simulink model "landing_model"  (R2025b)
settings: Solver=ode4  StartTime=0.0  StopTime=400  FixedStep=0.001  RelTol=1e-3
values from neighbouring files (symbols this model uses):
  a0 = 340.294    [basedata.m]    (also in basedata.mat; control_design.mat; landing_init.m; landing_plan.mat)
  b_ref = 2.0    (= 2)    [basedata.m]    (also in basedata.mat; control_design.mat; landing_init.m; landing_plan.mat)
  c_gear = [0.8e4, 1.4e4, 1.4e4]    [basedata.m]    (also in basedata.mat = [8000 14000 14000]; control_design.mat = [8000 14000 14000]; landing_init.m; landing_plan.mat = [8000 14000 14000])
  c_lat = [1.4e4, 2.2e4, 2.2e4]    [basedata.m]    (also in basedata.mat = [14000 22000 22000]; control_design.mat = [14000 22000 22000]; landing_init.m; landing_plan.mat = [14000 22000 22000])
  c_ref = 0.9    [basedata.m]    (also in basedata.mat; control_design.mat; landing_init.m; landing_plan.mat)
  c_roll = [0.020, 0.018, 0.018]    [basedata.m]    (also in basedata.mat = [0.02 0.018 0.018]; control_design.mat = [0.02 0.018 0.018]; landing_init.m; landing_plan.mat = [0.02 0.018 0.018])
  CD0 = 0.045    [basedata.m]    (also in basedata.mat; canshujisuan.m; control_design.mat; landing_init.m)
  CL0 = 0.083    [basedata.m]    (also in basedata.mat; control_design.mat; landing_init.m; landing_plan.mat)
  CLa = 3.80    (= 3.8)    [basedata.m]    (also in basedata.mat; canshujisuan.m = 2.5; control_design.mat; landing_init.m)
  Clb = -0.08    [basedata.m]    (also in basedata.mat; control_design.mat; landing_init.m; landing_plan.mat)
  Clda = -0.20    (= -0.2)    [basedata.m]    (also in basedata.mat; control_design.mat; landing_init.m; landing_plan.mat)
  CLde = 0.28    [basedata.m]    (also in basedata.mat; control_design.mat; landing_init.m; landing_plan.mat)
  Clp = -0.70    (= -0.7)    [basedata.m]    (also in basedata.mat; control_design.mat; landing_init.m; landing_plan.mat)
  CLq = 4.50    (= 4.5)    [basedata.m]    (also in basedata.mat; canshujisuan.m = 3; control_design.mat; landing_init.m)
  Clr = 0.08    [basedata.m]    (also in basedata.mat; control_design.mat; landing_init.m; landing_plan.mat)
  Cm0 = 0.060    (= 0.06)    [basedata.m]    (also in basedata.mat; control_design.mat; landing_init.m; landing_plan.mat)
  Cma = -0.80    (= -0.8)    [basedata.m]    (also in basedata.mat; control_design.mat; landing_init.m; landing_plan.mat)
  Cmde = -0.90    (= -0.9)    [basedata.m]    (also in basedata.mat; control_design.mat; landing_init.m; landing_plan.mat)
  Cmq = -18.0    (= -18)    [basedata.m]    (also in basedata.mat; control_design.mat; landing_init.m; landing_plan.mat)
  Cnb = 0.25    [basedata.m]    (also in basedata.mat; control_design.mat; landing_init.m; landing_plan.mat)
  Cndr = -0.15    [basedata.m]    (also in basedata.mat; control_design.mat; landing_init.m; landing_plan.mat)
  Cnp = -0.04    [basedata.m]    (also in basedata.mat; control_design.mat; landing_init.m; landing_plan.mat)
  Cnr = -0.45    [basedata.m]    (also in basedata.mat; control_design.mat; landing_init.m; landing_plan.mat)
  CSb = -0.70    (= -0.7)    [basedata.m]    (also in basedata.mat; control_design.mat; landing_init.m; landing_plan.mat)
  CSdr = 0.18    [basedata.m]    (also in basedata.mat; control_design.mat; landing_init.m; landing_plan.mat)
  CSr = 0.12    [basedata.m]    (also in basedata.mat; control_design.mat; landing_init.m; landing_plan.mat)
  D = 0.5 * rho0 * V^2 * S_ref * CD_current    [canshujisuan.m]
  D0 = 1400    [basedata.m]    (also in basedata.mat; control_design.mat; landing.m; landing_init.m)
  da_max = 25    [basedata.m]    (also in basedata.mat; control_design.mat; landing_init.m; landing_plan.mat)
  da_min = -da_max    (= -25)    [basedata.m]    (also in basedata.mat; control_design.mat; landing_init.m; landing_plan.mat)
  de_max = 25    [basedata.m]    (also in basedata.mat; control_design.mat; landing_init.m; landing_plan.mat)
  de_min = -de_max    (= -25)    [basedata.m]    (also in basedata.mat; control_design.mat; landing_init.m; landing_plan.mat)
  DH = pi / 180    (= 0.0174532925199)    [basedata.m]    (also in basedata.mat; control_design.mat; landing_init.m; landing_plan.mat)
  dr_max = 25    [basedata.m]    (also in basedata.mat; control_design.mat; landing_init.m; landing_plan.mat)
  dr_min = -dr_max    (= -25)    [basedata.m]    (also in basedata.mat; control_design.mat; landing_init.m; landing_plan.mat)
  g = 9.80665    [basedata.m]    (also in basedata.mat; canshujisuan.m; control_design.mat; landing_init.m)
  gamma1 = -0.125844364415    [basedata.mat]    (also in landing_trajectory.m = asin(max(min(gamma1_arg, 1), -1)); landingplan.mat)
  ground_z = 0.0    (= 0)    [basedata.m]    (also in basedata.mat; control_design.mat; landing_init.m; landing_plan.mat)
  HD = 180 / pi    (= 57.2957795131)    [basedata.m]    (also in basedata.mat; control_design.mat; landing_init.m; landing_plan.mat)
  I = [ Ixx, -Ixy, -Ixz ... (first row only)    [basedata.m]    (also in basedata.mat = [120  0  0; 0  480  0; 0  0  520]; control_design.mat = [120  0  0; 0  480  0; 0  0  520]; landing_init.m; landing_plan.mat = [120  0  0; 0  480  0; 0  0  520])
  K = 0.12    [basedata.m]    (also in basedata.mat; canshujisuan.m = 0.08; control_design.mat; landing_init.m)
  K_alpha = 7.5375    [basedata.mat]    (also in control_design.m = (((wd_pitch^2)-a24))/(2*kesi_pitch*wd_pitch); control_design.mat; controller.m = 5; landingplan.mat)
  K_beta = 10.5528846154    [basedata.mat]    (also in control_design.m = (((wd_yaw)^2)-b24)/(2*kesi_yaw*wd_yaw); control_design.mat; landingplan.mat)
  k_gear = [1.0e5, 3.0e5, 3.0e5]    [basedata.m]    (also in basedata.mat = [100000 300000 300000]; control_design.mat = [100000 300000 300000]; landing_init.m; landing_plan.mat = [100000 300000 300000])
  Kn_pitch = -0.120095403309    [basedata.mat]    (also in control_design.m = -(2.2*g*(wd_pitch)^2)/(Tr*(((wd_pitch)^2)-a24)*V_control*a34; control_design.mat; controller.m = (2.2*wd^2*g)/(Tr*(wd^2-a24)*V_test*a34); landingplan.mat)
  Kn_yaw = 0.435999267298    [basedata.mat]    (also in control_design.m = (2.2*g*wd_yaw^2)/(Tr_yaw*((wd_yaw^2)-b24)*V_control*b34); control_design.mat = -0.4656590814; landingplan.mat)
  Kw_pitch = -0.483749055178    [basedata.mat]    (also in control_design.m = -2*kesi_pitch*wd_pitch/a25; control_design.mat; controller.m = -(2*zeta*wd) / a25; landingplan.mat)
  Kw_yaw = -1.41496598639    [basedata.mat]    (also in control_design.m = -2*kesi_yaw*wd_yaw/b27; control_design.mat; landingplan.mat)
  m = 600.0    (= 600)    [basedata.m]    (also in basedata.mat; canshujisuan.m; control_design.mat; landing_init.m)
  mu_brake = [0.0, 0.55, 0.55]    [basedata.m]    (also in basedata.mat = [0 0.55 0.55]; control_design.mat = [0 0.55 0.55]; landing_init.m; landing_plan.mat = [0 0.55 0.55])
  phi0 = 0    [control_design.mat]    (also in landing.m; landing_init.m; landing_init.mat; landing_plan.mat)
  psi0 = 0    [control_design.mat]    (also in landing.m; landing_init.m; landing_init.mat; landing_plan.mat)
  r_left_b = r_gear_b(:,2)    [basedata.m]    (also in basedata.mat = [-0.333333333333 -0.8 0.65]; control_design.mat = [-0.333333333333 -0.8 0.65]; landing_init.m; landing_plan.mat = [-0.333333333333 -0.8 0.65])
  r_nose_b = r_gear_b(:,1)    [basedata.m]    (also in basedata.mat = [2 0 0.65]; control_design.mat = [2 0 0.65]; landing_init.m; landing_plan.mat = [2 0 0.65])
  r_right_b = r_gear_b(:,3)    [basedata.m]    (also in basedata.mat = [-0.333333333333 0.8 0.65]; control_design.mat = [-0.333333333333 0.8 0.65]; landing_init.m; landing_plan.mat = [-0.333333333333 0.8 0.65])
  rho0 = 1.225    [basedata.m]    (also in basedata.mat; canshujisuan.m; control_design.mat; landing_init.m)
  S_ref = 1.2    [basedata.m]    (also in basedata.mat; canshujisuan.m; control_design.mat; landing_init.m)
  theta0 = 0.0523560209424    [control_design.mat]    (also in landing.m = 0; landing_init.m; landing_init.mat = 0.0523598775598; landing_plan.mat)
  u0_b = 128    [control_design.mat]    (also in landing.m; landing_init.m; landing_init.mat = 100; landing_plan.mat)
  v0_b = 0    [control_design.mat]    (also in landing.m; landing_init.m; landing_init.mat; landing_plan.mat)
  v_eps = 0.20    (= 0.2)    [basedata.m]    (also in basedata.mat; control_design.mat; landing_init.m; landing_plan.mat)
  V_min = 3    [control_design.mat]    (also in landing.m; landing_init.m; landing_plan.mat; landingplan.mat)
  VR = 100    [basedata.m]    (also in basedata.mat; control_design.mat; landing.m; landing_init.m)
  w0_b = 0    [control_design.mat]    (also in landing.m; landing_init.m; landing_init.mat; landing_plan.mat)
  wheel_radius = 0.18    [basedata.m]    (also in basedata.mat; control_design.mat; landing_init.m; landing_plan.mat)
  WOW_on = 0.000    (= 0)    [basedata.m]    (also in basedata.mat; control_design.mat; landing_init.m; landing_plan.mat)
  Xg0 = -12000    [control_design.mat]    (also in landing.m; landing_init.m; landing_init.mat = -8000; landing_plan.mat)
  Yg0 = 0    [control_design.mat]    (also in landing.m; landing_init.m; landing_init.mat; landing_plan.mat)
  Zg0 = ground_z - wheel_radius - r_gear_b(3,1) + static_deflection    [basedata.m]    (also in basedata.mat = -0.8215943; control_design.mat = -1000; landing.m = -1000; landing_init.m = -1000)
undefined symbols (not defined in the file or in its folder): I_xz, I_yz, Ix_Iy, Iy_Iz, Iz_Ix
libraries: matrix_library x19, simulink x6, slpidlib x1
(part 2 of 3)

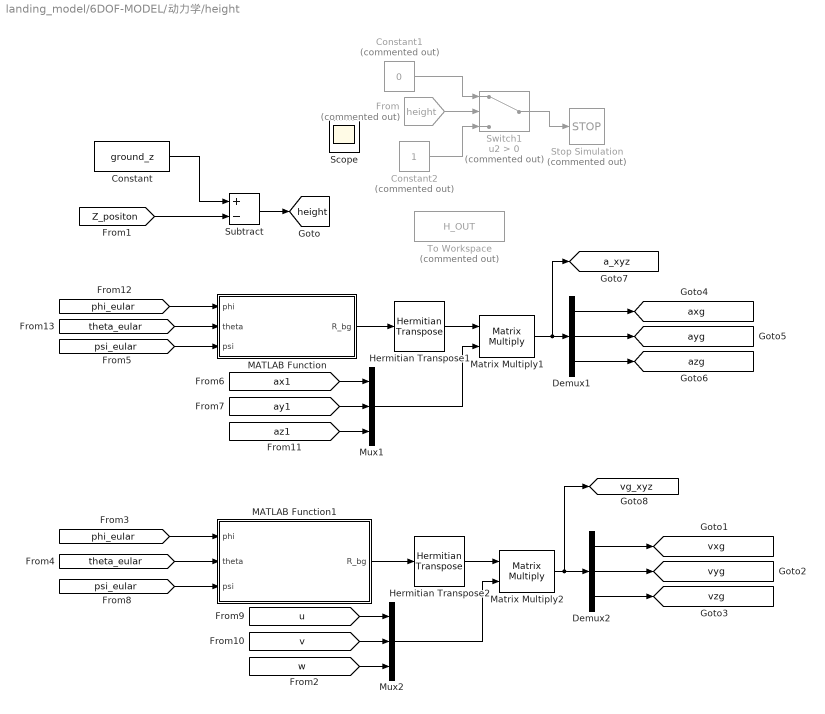
== system landing_model/6DOF-MODEL/动力学/height ==
  Constant : Constant  Value=ground_z
  Constant1 : Constant  Commented=on  Value=0
  Constant2 : Constant  Commented=on
  Demux1 : Demux  Outputs=3
  Demux2 : Demux  Outputs=3
  From : From  Commented=on  GotoTag=height  TagVisibility=global
  Hermitian Transpose1 : matrix_library/Hermitian Transpose
  Hermitian Transpose2 : matrix_library/Hermitian Transpose
  MATLAB Function : MATLAB Function  TreatAsAtomicUnit=on
  MATLAB Function1 : MATLAB Function  TreatAsAtomicUnit=on
  Matrix Multiply1 : Product  Multiplication=Matrix(*)
  Matrix Multiply2 : Product  Multiplication=Matrix(*)
  Mux1 : Mux  Inputs=3
  Mux2 : Mux  Inputs=3
  Scope : Scope
      settings: ActiveDisplayYMinimum=-1219.38221  ActiveDisplayYMaximum=10974.43988
  Stop Simulation : Stop  Commented=on
  Subtract : Sum  Inputs=+-
  Switch1 : Switch  Commented=on  Criteria=u2 > Threshold  SaturateOnIntegerOverflow=off  InputSameDT=off
  To Workspace : ToWorkspace  Commented=on  VariableName=H_OUT  SaveFormat=Timeseries  SampleTime=-1
  tag scope: a_xyz=global, axg=global, ayg=global, azg=global, height=global, vg_xyz=global, vxg=global, vyg=global, vzg=global
  wires:
  [ax1] -> Mux1/1
  [theta_eular] -> MATLAB Function/2(theta)
  MATLAB Function/1(R_bg) -> Hermitian Transpose1/1
  [psi_eular] -> MATLAB Function/3(psi)
  [ay1] -> Mux1/2
  Mux1/1 -> Matrix Multiply1/2
  [phi_eular] -> MATLAB Function/1(phi)
  Matrix Multiply1/1 -> [a_xyz], Demux1/1
  [az1] -> Mux1/3
  Demux1/3 -> [azg]
  Demux1/1 -> [axg]
  Demux1/2 -> [ayg]
  Hermitian Transpose1/1 -> Matrix Multiply1/1
  Switch1/1 -> Stop Simulation/1
  From/1 -> Switch1/2
  Constant1/1 -> Switch1/1
  Constant2/1 -> Switch1/3
  Demux2/2 -> [vyg]
  [u] -> Mux2/1
  Demux2/3 -> [vzg]
  [w] -> Mux2/3
  Mux2/1 -> Matrix Multiply2/2
  [phi_eular] -> MATLAB Function1/1(phi)
  Matrix Multiply2/1 -> [vg_xyz], Demux2/1
  Hermitian Transpose2/1 -> Matrix Multiply2/1
  [v] -> Mux2/2
  [theta_eular] -> MATLAB Function1/2(theta)
  [psi_eular] -> MATLAB Function1/3(psi)
  Demux2/1 -> [vxg]
  MATLAB Function1/1(R_bg) -> Hermitian Transpose2/1
  [Z_positon] -> Subtract/2
  Constant/1 -> Subtract/1
  Subtract/1 -> [height]

== system landing_model/6DOF-MODEL/动力学/rotation EQ ==
  L : Inport
  M : Inport  Port=2
  N : Inport  Port=3
  Constant : Constant  Value=I
  Demux : Demux  Outputs=3
  Display3 : Display
  Gain : Gain  Gain=inv(I)  Multiplication=Matrix(K*u) (u vector)
  Integrator : Integrator
  Integrator1 : Integrator
  Integrator2 : Integrator
  MATLAB Function1 : MATLAB Function  TreatAsAtomicUnit=on
  Mux : Mux  Inputs=3
  Mux1 : Mux  Inputs=3
  Product : Product  Inputs=3  Multiplication=Matrix(*)
  Reshape : Reshape  OutputDimensionality=Column vector (2-D)
  Reshape1 : Reshape
  Reshape2 : Reshape  OutputDimensionality=Column vector (2-D)
  Subsystem3 : Subsystem  Commented=on
  Sum : Sum  Inputs=|+-
  Sum1 : Sum  Inputs=|++
  p : Outport  VectorParamsAs1DForOutWhenUnconnected=off
  q : Outport  Port=2  VectorParamsAs1DForOutWhenUnconnected=off
  r : Outport  Port=3  VectorParamsAs1DForOutWhenUnconnected=off
  wires:
  Mux/1 -> Reshape/1, Display3/1
  Sum/1 -> Gain/1
  Demux/1 -> Integrator/1
  Demux/2 -> Integrator2/1
  Demux/3 -> Integrator1/1
  Gain/1 -> Reshape1/1
  Reshape1/1 -> Demux/1
  N/1 -> Mux/3
  L/1 -> Mux/1
  M/1 -> Mux/2
  Product/1 -> Sum/2
  MATLAB Function1/1(wB_X) -> Product/1
  Constant/1 -> Product/2
  Integrator/1 -> p/1, Mux1/1
  Integrator1/1 -> r/1, Mux1/3
  Integrator2/1 -> q/1, Mux1/2
  Reshape2/1 -> Product/3
  Mux1/1 -> Reshape2/1, MATLAB Function1/1(w)
  Reshape/1 -> Sum1/1
  [M_gear] -> Sum1/2
  Sum1/1 -> Sum/1

== system landing_model/6DOF-MODEL/动力学/姿态角 ==
  p : Inport
  q : Inport  Port=2
  r : Inport  Port=3
  Subsystem : Subsystem
  Subsystem1 : Subsystem
  Subsystem2 : Subsystem
  phi(eular) : Outport
  theta(eular) : Outport  Port=2
  psi(eular) : Outport  Port=3
  tag scope: phi_eular=global, psi_eular=global, theta_eular=global
  wires:
  q/1 -> Subsystem2/1(q), Subsystem1/1(q), Subsystem/2(q)
  Subsystem2/1(psi(euler)) -> [psi_eular], psi(eular)/1
  r/1 -> Subsystem2/2(r), Subsystem1/2(r), Subsystem/3(r)
  Subsystem/1(phi(euler)) -> Subsystem1/3(phi(euler)), Subsystem2/3(phi(euler)), phi(eular)/1, [phi_eular]
  Subsystem1/1(theta(euler)) -> Subsystem/4(theta(euler)), theta(eular)/1, [theta_eular], Subsystem2/4(theta(euler))
  p/1 -> Subsystem/1(p)

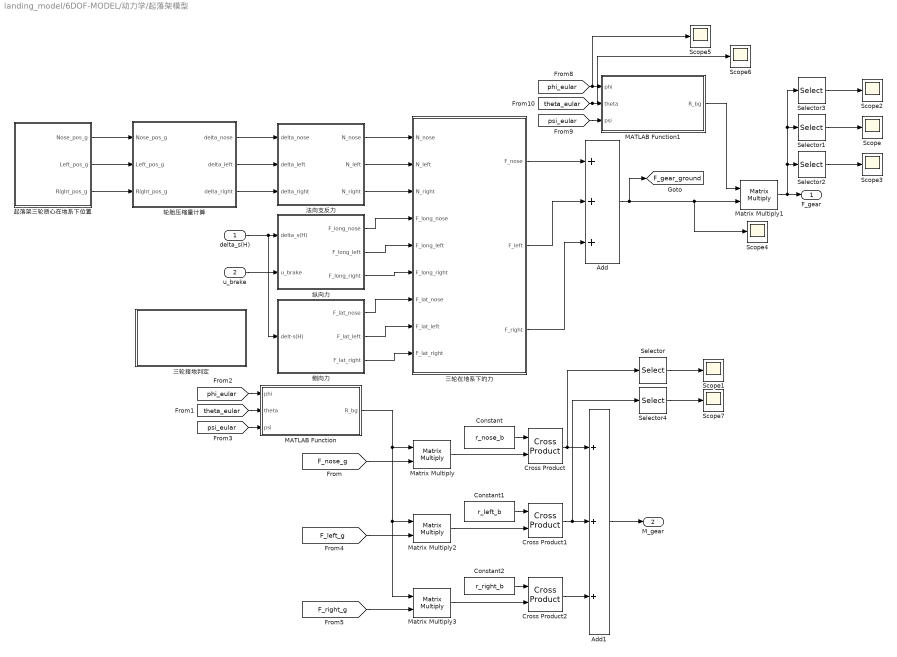
== system landing_model/6DOF-MODEL/动力学/起落架模型 ==
  delta_s(H) : Inport
  u_brake : Inport  Port=2
  Add : Sum  Inputs=+++
  Add1 : Sum  Inputs=+++
  Constant : Constant  Value=r_nose_b
  Constant1 : Constant  Value=r_left_b
  Constant2 : Constant  Value=r_right_b
  Cross Product : matrix_library/Cross Product
  Cross Product1 : matrix_library/Cross Product
  Cross Product2 : matrix_library/Cross Product
  MATLAB Function : MATLAB Function  TreatAsAtomicUnit=on
  MATLAB Function1 : MATLAB Function  TreatAsAtomicUnit=on
  Matrix Multiply{,1..3} (4 alike) : Product  Multiplication=Matrix(*)
  Scope{,1..7} (8 alike) : Scope
      Scope settings: ActiveDisplayYMinimum=-0.12099  ActiveDisplayYMaximum=0.34578  DataLoggingVariableName=ScopeData10
      Scope1 settings: ActiveDisplayYMinimum=-1  ActiveDisplayYMaximum=1  DataLoggingVariableName=ScopeData24
      Scope2 settings: ActiveDisplayYMinimum=-83.9341  ActiveDisplayYMaximum=93.97078
      Scope3 settings: ActiveDisplayYMinimum=-2.5669186787123E+8  ActiveDisplayYMaximum=5.7405258216679E+8  DataLoggingVariableName=ScopeData2
      Scope4 settings: ActiveDisplayYMinimum=-0.18022  ActiveDisplayYMaximum=0.17037  DataLoggingVariableName=ScopeData3
      Scope5 settings: ActiveDisplayYMinimum=1E-13  ActiveDisplayYMaximum=2.6E-13  DataLoggingVariableName=ScopeData4
      Scope6 settings: ActiveDisplayYMinimum=-1.96196  ActiveDisplayYMaximum=1.96294  DataLoggingVariableName=ScopeData5
      Scope7 settings: ActiveDisplayYMinimum=-973.30611  ActiveDisplayYMaximum=108.14512  DataLoggingVariableName=ScopeData4
  Selector : Selector  InputPortWidth=3  IndexOptions=Index vector (dialog)  Indices=3  OutputSizes=1
  Selector1 : Selector  InputPortWidth=3  IndexOptions=Index vector (dialog)  Indices=2  OutputSizes=1
  Selector2 : Selector  InputPortWidth=3  IndexOptions=Index vector (dialog)  Indices=3  OutputSizes=1
  Selector3 : Selector  InputPortWidth=3  IndexOptions=Index vector (dialog)  Indices=1  OutputSizes=1
  Selector4 : Selector  InputPortWidth=3  IndexOptions=Index vector (dialog)  Indices=3  OutputSizes=1
  三轮在地系下的力 : Subsystem
  三轮接地判定 : Subsystem
  侧向力 : Subsystem
  法向支反力 : Subsystem
  纵向力 : Subsystem
  起落架三轮质心在地系下位置 : Subsystem
  轮胎压缩量计算 : Subsystem
  F_gear : Outport
  M_gear : Outport  Port=2
  tag scope: F_gear_ground=global
  wires:
  起落架三轮质心在地系下位置/1(Nose_pos_g) -> 轮胎压缩量计算/1(Nose_pos_g)
  起落架三轮质心在地系下位置/2(Left_pos_g) -> 轮胎压缩量计算/2(Left_pos_g)
  起落架三轮质心在地系下位置/3(Right_pos_g) -> 轮胎压缩量计算/3(Right_pos_g)
  轮胎压缩量计算/1(delta_nose) -> 法向支反力/1(delta_nose)
  轮胎压缩量计算/2(delta_left) -> 法向支反力/2(delta_left)
  轮胎压缩量计算/3(delta_right) -> 法向支反力/3(delta_right)
  delta_s(H)/1 -> 侧向力/1(delt-s(H)), 纵向力/1(delta_s(H))
  u_brake/1 -> 纵向力/2(u_brake)
  法向支反力/1(N_nose) -> 三轮在地系下的力/1(N_nose)
  法向支反力/2(N_left) -> 三轮在地系下的力/2(N_left)
  法向支反力/3(N_right) -> 三轮在地系下的力/3(N_right)
  纵向力/1(F_long_nose) -> 三轮在地系下的力/4(F_long_nose)
  纵向力/2(F_long_left) -> 三轮在地系下的力/5(F_long_left)
  纵向力/3(F_long_right) -> 三轮在地系下的力/6(F_long_right)
  侧向力/1(F_lat_nose) -> 三轮在地系下的力/7(F_lat_nose)
  侧向力/2(F_lat_left) -> 三轮在地系下的力/8(F_lat_left)
  侧向力/3(F_lat_right) -> 三轮在地系下的力/9(F_lat_right)
  三轮在地系下的力/1(F_nose) -> Add/1
  三轮在地系下的力/2(F_left) -> Add/2
  三轮在地系下的力/3(F_right) -> Add/3
  Add/1 -> Scope4/1, Matrix Multiply1/2, [F_gear_ground]
  MATLAB Function1/1(R_bg) -> Matrix Multiply1/1
  [phi_eular] -> MATLAB Function1/1(phi), Scope5/1
  Matrix Multiply1/1 -> Selector3/1, Selector1/1, Selector2/1, F_gear/1
  Constant/1 -> Cross Product/1
  Constant1/1 -> Cross Product1/1
  Constant2/1 -> Cross Product2/1
  Cross Product/1 -> Add1/1, Selector/1
  Cross Product1/1 -> Selector4/1, Add1/2
  Cross Product2/1 -> Add1/3
  Add1/1 -> M_gear/1
  [theta_eular] -> Scope6/1, MATLAB Function1/2(theta)
  [psi_eular] -> MATLAB Function1/3(psi)
  [theta_eular] -> MATLAB Function/2(theta)
  [phi_eular] -> MATLAB Function/1(phi)
  [psi_eular] -> MATLAB Function/3(psi)
  MATLAB Function/1(R_bg) -> Matrix Multiply3/1, Matrix Multiply2/1, Matrix Multiply/1
  [F_nose_g] -> Matrix Multiply/2
  [F_right_g] -> Matrix Multiply3/2
  [F_left_g] -> Matrix Multiply2/2
  Matrix Multiply2/1 -> Cross Product1/2
  Matrix Multiply3/1 -> Cross Product2/2
  Matrix Multiply/1 -> Cross Product/2
  Selector1/1 -> Scope/1
  Selector3/1 -> Scope2/1
  Selector2/1 -> Scope3/1
  Selector/1 -> Scope1/1
  Selector4/1 -> Scope7/1

== system landing_model/control/俯仰通道/Subsystem ==
  Constant : Constant  Value=1000
  Constant1 : Constant  Value=0.001
  Gain : Gain  Gain=DH
  MATLAB Function : MATLAB Function  TreatAsAtomicUnit=on  SystemSampleTime=0.001
  Scope1 : Scope
      settings: ActiveDisplayYMinimum=-1.55977  ActiveDisplayYMaximum=22.25387  DataLoggingVariableName=ScopeData9
  h_cmd : Outport
  wires:
  Constant/1 -> MATLAB Function/1(H_target)
  MATLAB Function/1(hcmd) -> h_cmd/1, Scope1/1
  [Vg] -> MATLAB Function/2(Vg)
  [GAMMA_climb] -> Gain/1
  [start_fly] -> MATLAB Function/4(start_fly)
  Gain/1 -> MATLAB Function/3(gamma_climbmax)
  [Y_positon] -> MATLAB Function/5(H)
  Constant1/1 -> MATLAB Function/6(dt)

== system landing_model/control/俯仰通道/俯仰通道 ==
  nzc : Inport
  nz : Inport  Port=2
  q : Inport  Port=3
  Integrator : Integrator  ExternalReset=rising  LimitOutput=on  UpperSaturationLimit=25*DH  LowerSaturationLimit=-25*DH
  Ka : Constant  Value=K_alpha
  Kn : Constant  Value=Kn_pitch
  Kwy : Constant  Value=Kw_pitch
  Product : Product
  Product1 : Product
  Product2 : Product
  Scope : Scope  NumInputPorts=2
      settings: ActiveDisplayYMinimum=-1.37891  ActiveDisplayYMaximum=-0.78063
  Scope1 : Scope
      settings: ActiveDisplayYMinimum=-6.10633  ActiveDisplayYMaximum=5.39199  DataLoggingVariableName=ScopeData5
  Scope2 : Scope
      settings: ActiveDisplayYMinimum=-0.07148  ActiveDisplayYMaximum=0.49631  DataLoggingVariableName=ScopeData19
  Sum : Sum  Inputs=|+-
  Sum1 : Sum  Inputs=|+-
  Sum2 : Sum  Inputs=|+-
  伪攻角回路 : Subsystem
  delta_e : Outport
  wires:
  nz/1 -> Scope/2, Sum/2
  Sum/1 -> Product/2
  Product/1 -> Integrator/1
  Integrator/1 -> Scope2/1, Sum1/1
  Sum1/1 -> Product1/2
  Product1/1 -> Sum2/1
  Sum2/1 -> Product2/2
  Product2/1 -> Scope1/1, delta_e/1
  q/1 -> 伪攻角回路/1(q), Sum2/2
  伪攻角回路/1(alpha_c) -> Sum1/2
  Kn/1 -> Product/1
  Ka/1 -> Product1/1
  Kwy/1 -> Product2/1
  nzc/1 -> Scope/1, Sum/1
  [fly_height] -> Integrator/2

== system landing_model/control/俯仰通道/抬轮俯仰角控制通道 ==
  theta_cmd(H) : Inport
  K_theta : Gain  Gain=-0.3
  K_theta1 : Gain  Gain=0.8
  Scope : Scope
      settings: ActiveDisplayYMinimum=-32.03364  ActiveDisplayYMaximum=3.55929  DataLoggingVariableName=ScopeData4
  Sum : Sum  Inputs=|+-
  Sum1 : Sum  Inputs=+++
  de : Outport
  tag scope: theta_cmd=global
  wires:
  theta_cmd(H)/1 -> [theta_cmd], Sum/1
  [theta_eular] -> Sum/2
  K_theta/1 -> Sum1/1
  Sum/1 -> K_theta/1
  [q] -> K_theta1/1
  Sum1/1 -> de/1, Scope/1
  K_theta1/1 -> Sum1/2

== system landing_model/control/俯仰通道/高度控制 ==
  h_cmd : Inport
  Add1 : Sum
  Constant5 : Constant  Value=-1
  Cos : Trigonometry  Operator=cos
  Cos1 : Trigonometry  Operator=cos
  Divide : Product  Inputs=*/
  Gain1 : Gain  Gain=-0.05
  Gain7 : Gain  Gain=-0.005
  Product1 : Product
  Saturation : Saturate  UpperLimit=0  LowerLimit=-3
  Saturation1 : Saturate  UpperLimit=100  LowerLimit=-100
  Scope : Scope
      settings: ActiveDisplayYMinimum=-1.57089  ActiveDisplayYMaximum=-0.86886  DataLoggingVariableName=ScopeData11
  Scope1 : Scope  NumInputPorts=2
      settings: ActiveDisplayYMinimum=-118.65432  ActiveDisplayYMaximum=1076.1048  DataLoggingVariableName=ScopeData12
  Sum2 : Sum  Inputs=|+-
  Sum3 : Sum  Inputs=|++
  nzc : Outport
  wires:
  Gain7/1 -> Sum3/1
  [phi_eular] -> Cos/1
  Cos/1 -> Product1/1
  Product1/1 -> Divide/2
  Constant5/1 -> Divide/1
  [height] -> Scope1/2, Sum2/2
  Cos1/1 -> Product1/2
  [theta_eular] -> Cos1/1
  Sum3/1 -> Add1/1
  Gain1/1 -> Sum3/2
  Divide/1 -> Add1/2
  Add1/1 -> Scope/1, Saturation/1
  Saturation/1 -> nzc/1
  h_cmd/1 -> Scope1/1, Sum2/1
  [vzg] -> Gain1/1
  Sum2/1 -> Saturation1/1
  Saturation1/1 -> Gain7/1

== system landing_model/control/偏航通道/偏航通道三回路控制 ==
  nyc : Inport
  ny : Inport  Port=2
  r : Inport  Port=3
  Gain : Gain  Gain=Kn_yaw
  Gain1 : Gain  Gain=K_beta
  Gain2 : Gain  Gain=Kw_yaw
  Integrator : Integrator  ExternalReset=rising
  Scope : Scope  NumInputPorts=2
      settings: ActiveDisplayYMinimum=-0.013173747595067897  ActiveDisplayYMaximum=0.015707588107139965  DataLoggingVariableName=ScopeData20
  Scope1 : Scope
      settings: ActiveDisplayYMinimum=-0.125  ActiveDisplayYMaximum=1.125  DataLoggingVariableName=ScopeData3
  Sum : Sum  Inputs=|+-
  Sum1 : Sum  Inputs=|+-
  Sum2 : Sum  Inputs=|+-
  伪攻角回路 : Subsystem
  delta_r : Outport
  wires:
  ny/1 -> Sum/2, Scope/2
  nyc/1 -> Scope/1, Sum/1
  Gain/1 -> Integrator/1
  Integrator/1 -> Sum1/1
  Sum1/1 -> Gain1/1
  Gain1/1 -> Sum2/1
  r/1 -> 伪攻角回路/1(r), Sum2/2
  伪攻角回路/1(beta_c) -> Sum1/2
  Sum2/1 -> Gain2/1
  Sum/1 -> Gain/1
  [start_fly] -> Integrator/2, Scope1/1
  Gain2/1 -> delta_r/1

== system landing_model/control/偏航通道/偏航通道上升段控制 ==
  Add : Sum  Inputs=+++
  Constant1 : Constant  Value=0
  Constant2 : Constant  Value=0
  DivCrab : Product  Inputs=*/
  Gain : Gain  Gain=-1.5
  Gain1 : Gain  Gain=0.1
  Gain2 : Gain  Gain=-0.03
  Gain3 : Gain  Gain=0.5
  MaxVg2 : MinMax  Function=max  Inputs=2
  NegCrab : Gain  Gain=-1
  Scope1 : Scope
      settings: ActiveDisplayYMinimum=-0.78294447086433872  ActiveDisplayYMaximum=0.25366049676270425  DataLoggingVariableName=ScopeData6
  Scope2 : Scope
      settings: ActiveDisplayYMinimum=-0.7223173419510921  ActiveDisplayYMaximum=5.6358130379945655  DataLoggingVariableName=ScopeData10
  SelWy : Selector  IndexOptions=Index vector (dialog)  Indices=2  OutputSizes=1
  Sum1 : Sum  Inputs=+-+
  Sum3 : Sum  Inputs=|+-
  SumVygY : Sum
  Vmin3 : Constant  Value=3
  delta_r : Outport
  wires:
  Constant1/1 -> Sum3/1
  [Y_positon] -> Sum3/2, Scope2/1
  Sum3/1 -> Gain2/1
  Sum1/1 -> Gain/1
  [psi_eular] -> Sum1/2
  Constant2/1 -> Sum1/1
  Add/1 -> delta_r/1, Scope1/1
  [r] -> Gain3/1
  Gain/1 -> Add/2
  [Vwind_body] -> SelWy/1
  SelWy/1 -> DivCrab/1
  DivCrab/1 -> NegCrab/1
  [Vg] -> MaxVg2/1
  Vmin3/1 -> MaxVg2/2
  MaxVg2/1 -> DivCrab/2
  NegCrab/1 -> Sum1/3
  Gain3/1 -> Add/3
  [vyg] -> Gain1/1
  Gain2/1 -> SumVygY/1
  Gain1/1 -> SumVygY/2
  SumVygY/1 -> Add/1

== system landing_model/control/偏航通道/地面转向控制 ==
  Y_cmd : Inport
  Gain : Gain  Gain=-0.85
  K_z : Constant  Value=0.08
  KrGnd : Gain  Gain=-0.1
  Product : Product
  Saturation1 : Saturate  UpperLimit=25*DH  LowerLimit=-25*DH
  Scope : Scope
      settings: ActiveDisplayYMinimum=-508.96147  ActiveDisplayYMaximum=69.02503  DataLoggingVariableName=ScopeData17
  Scope1 : Scope
      settings: ActiveDisplayYMinimum=-0.01113  ActiveDisplayYMaximum=0.02225  DataLoggingVariableName=ScopeData18
  Scope2 : Scope
      settings: ActiveDisplayYMinimum=-0.18234993508252009  ActiveDisplayYMaximum=0.041149415742680995  DataLoggingVariableName=ScopeData12
  Sum : Sum  Inputs=|+-
  Sum1 : Sum  Inputs=+++
  delta_s(H) : Outport
  wires:
  Y_cmd/1 -> Sum/1
  [Y_positon] -> Scope/1, Sum/2
  [psi_eular] -> Gain/1
  Sum/1 -> Product/2
  K_z/1 -> Product/1
  Sum1/1 -> Saturation1/1
  Gain/1 -> Scope1/1, Sum1/2
  Product/1 -> Sum1/1
  Saturation1/1 -> Scope2/1, delta_s(H)/1
  [r] -> KrGnd/1
  KrGnd/1 -> Sum1/3

== system landing_model/control/偏航通道/航向过载指令 ==
  Add : Sum
  Gain2 : Gain  Gain=-0.001
  Gain3 : Gain  Gain=-0.5
  Scope1 : Scope
      settings: ActiveDisplayYMinimum=-0.49425  ActiveDisplayYMaximum=0.44405  DataLoggingVariableName=ScopeData7
  Scope2 : Scope
      settings: ActiveDisplayYMinimum=-0.0030373455421241311  ActiveDisplayYMaximum=0.0065428813537784592  DataLoggingVariableName=ScopeData8
  Scope3 : Scope
      settings: ActiveDisplayYMinimum=-125.58198  ActiveDisplayYMaximum=113.62326  DataLoggingVariableName=ScopeData5
  ny_cmd : Outport
  wires:
  Gain3/1 -> Add/2
  Add/1 -> ny_cmd/1, Scope2/1
  [Y_positon] -> Scope3/1, Gain2/1
  [psi_eular] -> Scope1/1, Gain3/1
  Gain2/1 -> Add/1

== system landing_model/control/滚转通道/Subsystem ==
  PHI_c : Inport
  P : Inport  Port=2
  phi : Inport  Port=3
  Gain1 : Gain  Gain=1/HD
  Integrator : Integrator
  Product : Product
  Product1 : Product
  Product2 : Product
  Scope : Scope  NumInputPorts=2
      settings: ActiveDisplayYMinimum=-0.0052080413702804192  ActiveDisplayYMaximum=0.0044166217070685382  DataLoggingVariableName=ScopeData2
  Sum : Sum  Inputs=|+-
  Sum1 : Sum  Inputs=|+-
  Sum2 : Sum  Inputs=|++
  kigamma_to_p : Constant  Value=0.5
  kp_to_da : Constant
  kphi_to_wx : Constant  Value=50
  da : Outport
  wires:
  PHI_c/1 -> Gain1/1
  Sum/1 -> Product/2, Product2/2
  Sum1/1 -> Product1/2
  Product1/1 -> da/1
  P/1 -> Sum1/2
  phi/1 -> Scope/2, Sum/2
  kigamma_to_p/1 -> Product2/1
  Product2/1 -> Integrator/1
  Product/1 -> Sum2/1
  Sum2/1 -> Sum1/1
  Integrator/1 -> Sum2/2
  Gain1/1 -> Scope/1, Sum/1
  kphi_to_wx/1 -> Product/1
  kp_to_da/1 -> Product1/1

== system landing_model/control/滚转通道/Subsystem1 ==
  Constant : Constant  Value=0
  Gain : Gain  Gain=1.5
  Gain1 : Gain  Gain=0.8
  Scope : Scope  NumInputPorts=2
      settings: ActiveDisplayYMinimum=-0.0052080413702804192  ActiveDisplayYMaximum=0.0044166217070685382  DataLoggingVariableName=ScopeData5
  Sum : Sum  Inputs=|+-
  Sum1 : Sum  Inputs=|+-
  da : Outport
  wires:
  Sum1/1 -> da/1
  Gain/1 -> Sum1/1
  Sum/1 -> Gain/1
  [p] -> Gain1/1
  Constant/1 -> Sum/1, Scope/1
  Gain1/1 -> Sum1/2
  [phi_eular] -> Sum/2, Scope/2

== system landing_model/6DOF-MODEL/AERO-PARAMETER/无量纲化角速率/Subsystem ==
  r : Inport
  Va : Inport  Port=2
  Constant4 : Constant  Value=b_ref
  Divide : Product  Inputs=*/
  Gain : Gain  Gain=2
  Product : Product
  r_hat : Outport
  wires:
  Va/1 -> Gain/1
  r/1 -> Product/1
  Constant4/1 -> Product/2
  Product/1 -> Divide/1
  Divide/1 -> r_hat/1
  Gain/1 -> Divide/2

== system landing_model/6DOF-MODEL/AERO-PARAMETER/无量纲化角速率/Subsystem1 ==
  q : Inport
  Va : Inport  Port=2
  Constant4 : Constant  Value=c_ref
  Divide : Product  Inputs=*/
  Gain : Gain  Gain=2
  Product : Product
  Scope : Scope
      settings: ActiveDisplayYMinimum=-0.16355  ActiveDisplayYMaximum=0.33012  DataLoggingVariableName=ScopeData22
  q_hat : Outport
  wires:
  Va/1 -> Gain/1
  q/1 -> Scope/1, Product/1
  Constant4/1 -> Product/2
  Product/1 -> Divide/1
  Divide/1 -> q_hat/1
  Gain/1 -> Divide/2

== system landing_model/6DOF-MODEL/AERO-PARAMETER/无量纲化角速率/Subsystem2 ==
  p : Inport
  Va : Inport  Port=2
  Constant4 : Constant  Value=b_ref
  Divide : Product  Inputs=*/
  Gain : Gain  Gain=2
  Product : Product
  p_hat : Outport
  wires:
  Va/1 -> Gain/1
  p/1 -> Product/1
  Constant4/1 -> Product/2
  Product/1 -> Divide/1
  Divide/1 -> p_hat/1
  Gain/1 -> Divide/2

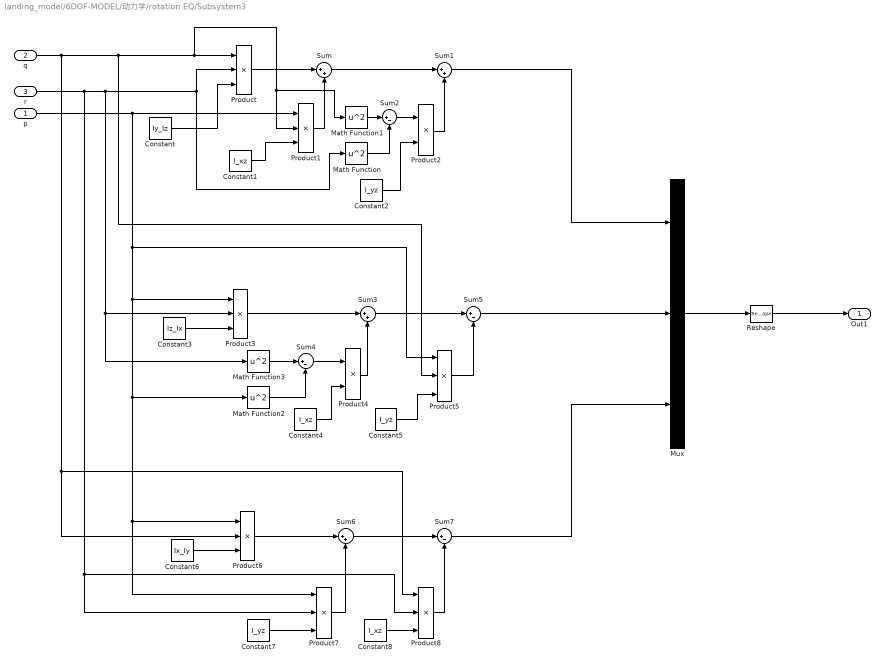
== system landing_model/6DOF-MODEL/动力学/rotation EQ/Subsystem3 ==
  p : Inport
  q : Inport  Port=2
  r : Inport  Port=3
  Constant : Constant  Value=Iy_Iz
  Constant1 : Constant  Value=I_xz
  Constant2 : Constant  Value=I_yz
  Constant3 : Constant  Value=Iz_Ix
  Constant4 : Constant  Value=I_xz
  Constant5 : Constant  Value=I_yz
  Constant6 : Constant  Value=Ix_Iy
  Constant7 : Constant  Value=I_yz
  Constant8 : Constant  Value=I_xz
  Math Function{,1..3} (4 alike) : Math  Operator=square
  Mux : Mux  Inputs=3
  Product{,1,3,5..8} (7 alike) : Product  Inputs=3
  Product2 : Product
  Product4 : Product
  Reshape : Reshape  OutputDimensionality=Column vector (2-D)
  Sum{,1,3,6} (4 alike) : Sum  Inputs=|++
  Sum{2,4..5,7} (4 alike) : Sum  Inputs=|+-
  Out1 : Outport
  wires:
  q/1 -> Product8/1, Product6/2, Product5/2, Math Function1/1, Product1/2, Product/1
  r/1 -> Product8/2, Product7/2, Math Function3/1, Product3/2, Math Function/1, Product/2
  Constant/1 -> Product/3
  Product/1 -> Sum/1
  Constant1/1 -> Product1/3
  p/1 -> Product7/1, Product6/1, Math Function2/1, Product3/1, Product5/1, Product1/1
  Product1/1 -> Sum/2
  Sum/1 -> Sum1/1
  Product2/1 -> Sum1/2
  Constant2/1 -> Product2/2
  Sum2/1 -> Product2/1
  Math Function1/1 -> Sum2/1
  Math Function/1 -> Sum2/2
  Constant3/1 -> Product3/3
  Product3/1 -> Sum3/1
  Math Function3/1 -> Sum4/1
  Math Function2/1 -> Sum4/2
  Sum4/1 -> Product4/1
  Product4/1 -> Sum3/2
  Constant4/1 -> Product4/2
  Sum3/1 -> Sum5/1
  Product5/1 -> Sum5/2
  Constant5/1 -> Product5/3
  Constant6/1 -> Product6/3
  Product6/1 -> Sum6/1
  Constant7/1 -> Product7/3
  Product7/1 -> Sum6/2
  Sum6/1 -> Sum7/1
  Product8/1 -> Sum7/2
  Constant8/1 -> Product8/3
  Sum5/1 -> Mux/2
  Sum1/1 -> Mux/1
  Sum7/1 -> Mux/3
  Mux/1 -> Reshape/1
  Reshape/1 -> Out1/1

== system landing_model/6DOF-MODEL/动力学/姿态角/Subsystem ==
  p : Inport
  q : Inport  Port=2
  r : Inport  Port=3
  theta(euler) : Inport  Port=4
  Integrator : Integrator  InitialCondition=phi0
  Product : Product  Inputs=3
  Product1 : Product  Inputs=3
  Sum : Sum  Inputs=|++
  Sum1 : Sum  Inputs=|++
  Trigonometric Function : Trigonometry
  Trigonometric Function1 : Trigonometry  Operator=tan
  Trigonometric Function2 : Trigonometry  Operator=cos
  Trigonometric Function3 : Trigonometry  Operator=tan
  phi(euler) : Outport
  wires:
  p/1 -> Sum/1
  Trigonometric Function1/1 -> Product/3
  q/1 -> Product/1
  Trigonometric Function/1 -> Product/2
  theta(euler)/1 -> Trigonometric Function3/1, Trigonometric Function1/1
  Product/1 -> Sum/2
  Sum/1 -> Sum1/1
  r/1 -> Product1/1
  Trigonometric Function2/1 -> Product1/2
  Trigonometric Function3/1 -> Product1/3
  Product1/1 -> Sum1/2
  Sum1/1 -> Integrator/1  "phi_dot"
  Integrator/1 -> Trigonometric Function2/1, Trigonometric Function/1, phi(euler)/1

== system landing_model/6DOF-MODEL/动力学/姿态角/Subsystem1 ==
  q : Inport
  r : Inport  Port=2
  phi(euler) : Inport  Port=3
  Integrator : Integrator  InitialCondition=theta0
  Product : Product
  Product1 : Product
  Sum : Sum  Inputs=|+-
  Trigonometric Function : Trigonometry  Operator=cos
  Trigonometric Function1 : Trigonometry
  theta(euler) : Outport
  wires:
  q/1 -> Product/1
  phi(euler)/1 -> Trigonometric Function1/1, Trigonometric Function/1
  Trigonometric Function/1 -> Product/2
  Product/1 -> Sum/1
  r/1 -> Product1/1
  Trigonometric Function1/1 -> Product1/2
  Product1/1 -> Sum/2
  Sum/1 -> Integrator/1  "theta_dot"
  Integrator/1 -> theta(euler)/1

== system landing_model/6DOF-MODEL/动力学/姿态角/Subsystem2 ==
  q : Inport
  r : Inport  Port=2
  phi(euler) : Inport  Port=3
  theta(euler) : Inport  Port=4
  Integrator : Integrator  InitialCondition=psi0
  Product : Product  Inputs=**/
  Product1 : Product  Inputs=**/
  Sum : Sum  Inputs=|++
  Trigonometric Function : Trigonometry
  Trigonometric Function1 : Trigonometry  Operator=cos
  Trigonometric Function2 : Trigonometry  Operator=cos
  Trigonometric Function3 : Trigonometry  Operator=cos
  psi(euler) : Outport
  wires:
  q/1 -> Product/1
  phi(euler)/1 -> Trigonometric Function2/1, Trigonometric Function/1
  Trigonometric Function/1 -> Product/2
  theta(euler)/1 -> Trigonometric Function1/1, Trigonometric Function3/1
  Trigonometric Function1/1 -> Product/3
  Product/1 -> Sum/1
  r/1 -> Product1/1
  Trigonometric Function2/1 -> Product1/2
  Trigonometric Function3/1 -> Product1/3
  Product1/1 -> Sum/2
  Sum/1 -> Integrator/1  "psi_dot"
  Integrator/1 -> psi(euler)/1

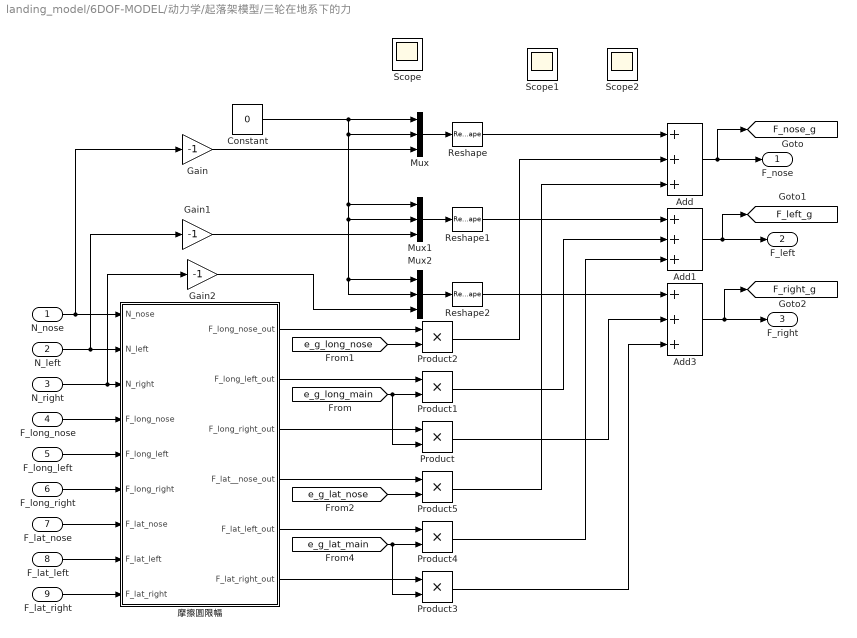
== system landing_model/6DOF-MODEL/动力学/起落架模型/三轮在地系下的力 ==
  N_nose : Inport
  N_left : Inport  Port=2
  N_right : Inport  Port=3
  F_long_nose : Inport  Port=4
  F_long_left : Inport  Port=5
  F_long_right : Inport  Port=6
  F_lat_nose : Inport  Port=7
  F_lat_left : Inport  Port=8
  F_lat_right : Inport  Port=9
  Add : Sum  Inputs=+++
  Add1 : Sum  Inputs=+++
  Add3 : Sum  Inputs=+++
  Constant : Constant  Value=0
  Gain : Gain  Gain=-1
  Gain1 : Gain  Gain=-1
  Gain2 : Gain  Gain=-1
  Mux : Mux  Inputs=3
  Mux1 : Mux  Inputs=3
  Mux2 : Mux  Inputs=3
  Product{,1..5} (6 alike) : Product
  Reshape : Reshape  OutputDimensionality=Column vector (2-D)
  Reshape1 : Reshape  OutputDimensionality=Column vector (2-D)
  Reshape2 : Reshape  OutputDimensionality=Column vector (2-D)
  Scope : Scope
      settings: ActiveDisplayYMinimum=-1  ActiveDisplayYMaximum=1  DataLoggingVariableName=ScopeData12
  Scope1 : Scope
      settings: ActiveDisplayYMinimum=-3888.85928  ActiveDisplayYMaximum=34999.73355  DataLoggingVariableName=ScopeData13
  Scope2 : Scope
      settings: ActiveDisplayYMinimum=-1  ActiveDisplayYMaximum=1  DataLoggingVariableName=ScopeData14
  摩擦圆限幅 : Subsystem
  F_nose : Outport
  F_left : Outport  Port=2
  F_right : Outport  Port=3
  tag scope: F_left_g=global, F_nose_g=global, F_right_g=global
  wires:
  Product1/1 -> Add1/2
  Constant/1 -> Mux1/2, Mux2/1, Mux2/2, Mux1/1, Mux/2, Mux/1
  [e_g_long_nose] -> Product2/2
  [e_g_long_main] -> Product/2, Product1/2
  Product5/1 -> Add/3
  Product2/1 -> Add/2
  Product/1 -> Add3/2
  [e_g_lat_nose] -> Product5/2
  [e_g_lat_main] -> Product3/2, Product4/2
  Product4/1 -> Add1/3
  Product3/1 -> Add3/3
  Add/1 -> [F_nose_g], F_nose/1
  Add1/1 -> [F_left_g], F_left/1
  Add3/1 -> [F_right_g], F_right/1
  Mux/1 -> Reshape/1
  Mux2/1 -> Reshape2/1
  Reshape2/1 -> Add3/1
  Reshape1/1 -> Add1/1
  Mux1/1 -> Reshape1/1
  Reshape/1 -> Add/1
  F_long_nose/1 -> 摩擦圆限幅/4(F_long_nose)
  F_long_left/1 -> 摩擦圆限幅/5(F_long_left)
  F_long_right/1 -> 摩擦圆限幅/6(F_long_right)
  F_lat_nose/1 -> 摩擦圆限幅/7(F_lat_nose)
  F_lat_left/1 -> 摩擦圆限幅/8(F_lat_left)
  F_lat_right/1 -> 摩擦圆限幅/9(F_lat_right)
  摩擦圆限幅/1(F_long_nose_out) -> Product2/1
  摩擦圆限幅/4(F_lat__nose_out) -> Product5/1
  摩擦圆限幅/2(F_long_left_out) -> Product1/1
  摩擦圆限幅/5(F_lat_left_out) -> Product4/1
  摩擦圆限幅/3(F_long_right_out) -> Product/1
  摩擦圆限幅/6(F_lat_right_out) -> Product3/1
  N_nose/1 -> Gain/1, 摩擦圆限幅/1(N_nose)
  N_left/1 -> Gain1/1, 摩擦圆限幅/2(N_left)
  N_right/1 -> Gain2/1, 摩擦圆限幅/3(N_right)
  Gain/1 -> Mux/3
  Gain1/1 -> Mux1/3
  Gain2/1 -> Mux2/3

== system landing_model/6DOF-MODEL/动力学/起落架模型/三轮接地判定 ==
  Logical Operator : Logic  AllPortsSameDT=off  OutDataTypeStr=boolean
  Logical Operator1 : Logic  Operator=NOR  Inputs=3  AllPortsSameDT=off  OutDataTypeStr=boolean
  tag scope: contact_main=global, no_contact=global
  wires:
  Logical Operator/1 -> [contact_main]
  [contact_nose] -> Logical Operator1/1
  [contact_left] -> Logical Operator1/2, Logical Operator/1
  [contact_right] -> Logical Operator1/3, Logical Operator/2
  Logical Operator1/1 -> [no_contact]

== system landing_model/6DOF-MODEL/动力学/起落架模型/侧向力 ==
  delt-s(H) : Inport
  Constant : Constant  Value=c_lat
  Demux : Demux  Outputs=3
  Gain : Gain  Gain=-1
  Gain1 : Gain  Gain=-1
  Gain2 : Gain  Gain=-1
  Product : Product
  Product1 : Product
  Product2 : Product
  Subsystem : Subsystem
  Subsystem1 : Subsystem
  Subsystem2 : Subsystem
  Subsystem3 : Subsystem
  F_lat_nose : Outport
  F_lat_left : Outport  Port=2
  F_lat_right : Outport  Port=3
  wires:
  delt-s(H)/1 -> Subsystem/1(delt-s(H))
  Constant/1 -> Demux/1
  Subsystem/1(V_lat_nose) -> Product/1
  Demux/1 -> Product/2
  Subsystem/2(V_lat_left) -> Product1/1
  Subsystem/3(V_lat_right) -> Product2/1
  Demux/2 -> Product1/2
  Demux/3 -> Product2/2
  Product/1 -> Gain/1
  Product1/1 -> Gain1/1
  Product2/1 -> Gain2/1
  Gain/1 -> Subsystem2/1(In1)
  Subsystem2/1(F_lat_nose) -> F_lat_nose/1
  Gain1/1 -> Subsystem1/1(In1)
  Subsystem1/1(F_lat_left) -> F_lat_left/1
  Gain2/1 -> Subsystem3/1(In1)
  Subsystem3/1(F_lat_right) -> F_lat_right/1

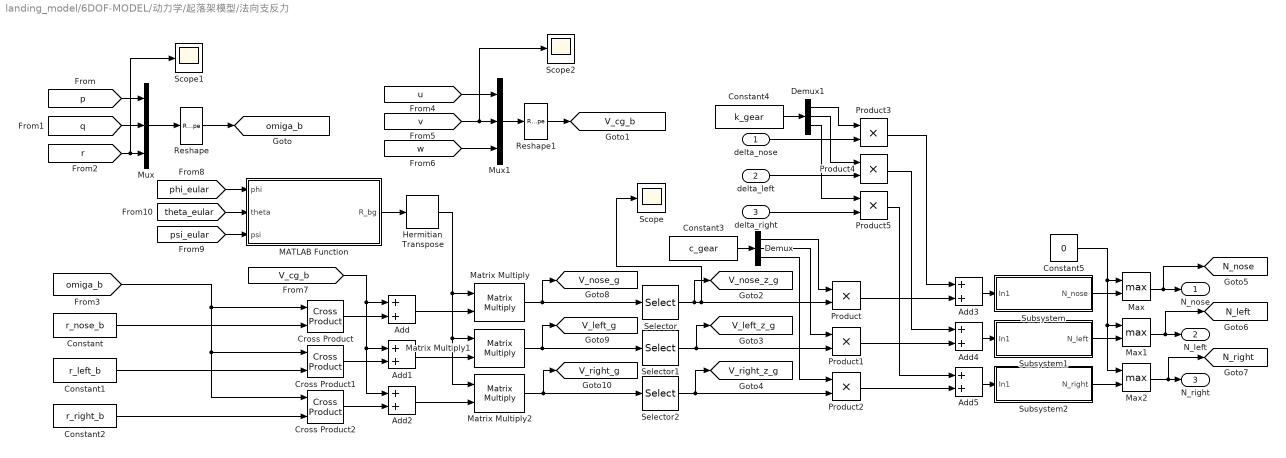
== system landing_model/6DOF-MODEL/动力学/起落架模型/法向支反力 ==
  delta_nose : Inport
  delta_left : Inport  Port=2
  delta_right : Inport  Port=3
  Add{,1..5} (6 alike) : Sum
  Constant : Constant  Value=r_nose_b
  Constant1 : Constant  Value=r_left_b
  Constant2 : Constant  Value=r_right_b
  Constant3 : Constant  Value=c_gear
  Constant4 : Constant  Value=k_gear
  Constant5 : Constant  Value=0
  Cross Product : matrix_library/Cross Product
  Cross Product1 : matrix_library/Cross Product
  Cross Product2 : matrix_library/Cross Product
  Demux : Demux  Outputs=3
  Demux1 : Demux  Outputs=3
  Hermitian Transpose : matrix_library/Hermitian Transpose
  MATLAB Function : MATLAB Function  TreatAsAtomicUnit=on
  Matrix Multiply : Product  Multiplication=Matrix(*)
  Matrix Multiply1 : Product  Multiplication=Matrix(*)
  Matrix Multiply2 : Product  Multiplication=Matrix(*)
  Max : MinMax  Function=max  Inputs=2
  Max1 : MinMax  Function=max  Inputs=2
  Max2 : MinMax  Function=max  Inputs=2
  Mux : Mux  Inputs=3
  Mux1 : Mux  Inputs=3
  Product{,1..5} (6 alike) : Product
  Reshape : Reshape  OutputDimensionality=Column vector (2-D)
  Reshape1 : Reshape  OutputDimensionality=Column vector (2-D)
  Scope : Scope
      settings: ActiveDisplayYMinimum=-2180.07321  ActiveDisplayYMaximum=4700.49414  DataLoggingVariableName=ScopeData15
  Scope1 : Scope
      settings: ActiveDisplayYMinimum=-2.3E-16  ActiveDisplayYMaximum=4.2E-16  DataLoggingVariableName=ScopeData16
  Scope2 : Scope
      settings: ActiveDisplayYMinimum=-8E-8  ActiveDisplayYMaximum=6.8E-7  DataLoggingVariableName=ScopeData17
  Selector : Selector  InputPortWidth=3  IndexOptions=Index vector (dialog)  Indices=3  OutputSizes=1
  Selector1 : Selector  InputPortWidth=3  IndexOptions=Index vector (dialog)  Indices=3  OutputSizes=1
  Selector2 : Selector  InputPortWidth=3  IndexOptions=Index vector (dialog)  Indices=3  OutputSizes=1
  Subsystem : Subsystem
  Subsystem1 : Subsystem
  Subsystem2 : Subsystem
  N_nose : Outport
  N_left : Outport  Port=2
  N_right : Outport  Port=3
  tag scope: N_left=global, N_nose=global, N_right=global, V_cg_b=global, V_left_g=global, V_left_z_g=global, V_nose_g=global, V_nose_z_g=global, V_right_g=global, V_right_z_g=global, omiga_b=global
  wires:
  [p] -> Mux/1
  [r] -> Scope1/1, Mux/3
  [q] -> Mux/2
  Mux/1 -> Reshape/1
  Reshape/1 -> [omiga_b]
  Constant2/1 -> Cross Product2/2
  Constant1/1 -> Cross Product1/2
  Constant/1 -> Cross Product/2
  [omiga_b] -> Cross Product1/1, Cross Product2/1, Cross Product/1
  [v] -> Scope2/1, Mux1/2
  [u] -> Mux1/1
  [w] -> Mux1/3
  Mux1/1 -> Reshape1/1
  Reshape1/1 -> [V_cg_b]
  Cross Product/1 -> Add/2
  Cross Product1/1 -> Add1/2
  Cross Product2/1 -> Add2/2
  [V_cg_b] -> Add/1, Add1/1, Add2/1
  MATLAB Function/1(R_bg) -> Hermitian Transpose/1
  [phi_eular] -> MATLAB Function/1(phi)
  Add1/1 -> Matrix Multiply1/2
  Add2/1 -> Matrix Multiply2/2
  Add/1 -> Matrix Multiply/2
  Hermitian Transpose/1 -> Matrix Multiply/1, Matrix Multiply1/1, Matrix Multiply2/1
  Matrix Multiply/1 -> [V_nose_g], Selector/1
  Matrix Multiply1/1 -> [V_left_g], Selector1/1
  Matrix Multiply2/1 -> [V_right_g], Selector2/1
  Product/1 -> Add3/2
  Product3/1 -> Add3/1
  Product1/1 -> Add4/2
  Product2/1 -> Add5/2
  Product4/1 -> Add4/1
  Product5/1 -> Add5/1
  Add4/1 -> Subsystem1/1(In1)
  Add5/1 -> Subsystem2/1(In1)
  delta_nose/1 -> Product3/2
  delta_left/1 -> Product4/2
  delta_right/1 -> Product5/2
  Selector/1 -> Product/2, Scope/1, [V_nose_z_g]
  Selector1/1 -> Product1/2, [V_left_z_g]
  Selector2/1 -> Product2/2, [V_right_z_g]
  [theta_eular] -> MATLAB Function/2(theta)
  [psi_eular] -> MATLAB Function/3(psi)
  Constant3/1 -> Demux/1
  Demux/1 -> Product/1
  Demux/3 -> Product2/1
  Constant4/1 -> Demux1/1
  Demux1/1 -> Product3/1
  Demux1/2 -> Product4/1
  Demux1/3 -> Product5/1
  Add3/1 -> Subsystem/1(In1)
  Max/1 -> [N_nose], N_nose/1
  Subsystem1/1(N_left) -> Max1/2
  Max1/1 -> [N_left], N_left/1
  Subsystem/1(N_nose) -> Max/2
  Subsystem2/1(N_right) -> Max2/2
  Max2/1 -> [N_right], N_right/1
  Constant5/1 -> Max2/1, Max1/1, Max/1
  Demux/2 -> Product1/1

== system landing_model/6DOF-MODEL/动力学/起落架模型/纵向力 ==
  delta_s(H) : Inport
  u_brake : Inport  Port=2
  Subsystem : Subsystem
  Subsystem1 : Subsystem
  F_long_nose : Outport
  F_long_left : Outport  Port=2
  F_long_right : Outport  Port=3
  wires:
  delta_s(H)/1 -> Subsystem/1(delt-s(H))
  Subsystem/1(V_long_nose) -> Subsystem1/1(V_long_nose)
  Subsystem/2(V_long_left) -> Subsystem1/2(V_long_left)
  Subsystem/3(V_long_right) -> Subsystem1/3(V_long_right)
  u_brake/1 -> Subsystem1/4(u_brake)
  Subsystem1/1(F_long_nose) -> F_long_nose/1
  Subsystem1/2(F_long_left) -> F_long_left/1
  Subsystem1/3(F_long_right) -> F_long_right/1

== system landing_model/6DOF-MODEL/动力学/起落架模型/起落架三轮质心在地系下位置 ==
  Add : Sum
  Add1 : Sum
  Add2 : Sum
  Constant : Constant  Value=r_nose_b
  Constant1 : Constant  Value=r_left_b
  Constant2 : Constant  Value=r_right_b
  MATLAB Function : MATLAB Function  TreatAsAtomicUnit=on
  Matrix Multiply : Product  Multiplication=Matrix(*)
  Matrix Multiply1 : Product  Multiplication=Matrix(*)
  Matrix Multiply2 : Product  Multiplication=Matrix(*)
  Mux : Mux  Inputs=3
  Scope : Scope
      settings: ActiveDisplayYMinimum=0.171594249  ActiveDisplayYMaximum=0.171594306  DataLoggingVariableName=ScopeData9
  Scope1 : Scope
      settings: ActiveDisplayYMinimum=-125.58198  ActiveDisplayYMaximum=113.62326  DataLoggingVariableName=ScopeData18
  Scope2 : Scope
      settings: ActiveDisplayYMinimum=-3.83794  ActiveDisplayYMaximum=0.42644  DataLoggingVariableName=ScopeData19
  Selector : Selector  InputPortWidth=3  IndexOptions=Index vector (dialog)  Indices=2  OutputSizes=1
  Transpose : matrix_library/Transpose
  Nose_pos_g : Outport
  Left_pos_g : Outport  Port=2
  Right_pos_g : Outport  Port=3
  tag scope: Left_pos_g=global, Nose_position_g=global, Right_pos_g=global
  wires:
  Constant1/1 -> Matrix Multiply1/2
  Transpose/1 -> Matrix Multiply2/1, Matrix Multiply1/1, Matrix Multiply/1
  [psi_eular] -> MATLAB Function/3(psi)
  [phi_eular] -> MATLAB Function/1(phi), Scope2/1
  Constant2/1 -> Matrix Multiply2/2
  Matrix Multiply1/1 -> Add1/2
  Constant/1 -> Matrix Multiply/2
  [theta_eular] -> MATLAB Function/2(theta)
  MATLAB Function/1(R_bg) -> Transpose/1
  Matrix Multiply/1 -> Add/2
  Matrix Multiply2/1 -> Add2/2
  [Z_positon] -> Mux/3
  [Y_positon] -> Scope1/1, Mux/2
  [X_positon] -> Mux/1
  Mux/1 -> Add/1, Add1/1, Add2/1
  Add/1 -> Selector/1, Nose_pos_g/1, [Nose_position_g]
  Add1/1 -> Left_pos_g/1, [Left_pos_g]
  Add2/1 -> Right_pos_g/1, [Right_pos_g]
  Selector/1 -> Scope/1

== system landing_model/6DOF-MODEL/动力学/起落架模型/轮胎压缩量计算 ==
  Nose_pos_g : Inport
  Left_pos_g : Inport  Port=2
  Right_pos_g : Inport  Port=3
  Constant : Constant  Value=wheel_radius
  Constant1 : Constant  Value=ground_z
  Constant2 : Constant  Value=0
  Constant4 : Constant
  Saturation : Saturate  UpperLimit=wheel_radius  LowerLimit=0
  Saturation1 : Saturate  UpperLimit=wheel_radius  LowerLimit=0
  Saturation2 : Saturate  UpperLimit=wheel_radius  LowerLimit=0
  Scope : Scope
      settings: ActiveDisplayYMinimum=-0.0225  ActiveDisplayYMaximum=0.2025  DataLoggingVariableName=ScopeData11
  Scope1 : Scope
      settings: ActiveDisplayYMinimum=-0.0225  ActiveDisplayYMaximum=0.2025  DataLoggingVariableName=ScopeData3
  Selector : Selector  InputPortWidth=3  IndexOptions=Index vector (dialog)  Indices=3  OutputSizes=1
  Selector1 : Selector  InputPortWidth=3  IndexOptions=Index vector (dialog)  Indices=3  OutputSizes=1
  Selector2 : Selector  InputPortWidth=3  IndexOptions=Index vector (dialog)  Indices=3  OutputSizes=1
  Subtract{,1..5} (6 alike) : Sum  Inputs=+-
  Switch3 : Switch  Criteria=u2 > Threshold  Threshold=WOW_on  SaturateOnIntegerOverflow=off  InputSameDT=off
  Switch4 : Switch  Criteria=u2 > Threshold  Threshold=WOW_on  SaturateOnIntegerOverflow=off  InputSameDT=off
  Switch5 : Switch  Criteria=u2 > Threshold  Threshold=WOW_on  SaturateOnIntegerOverflow=off  InputSameDT=off
  delta_nose : Outport
  delta_left : Outport  Port=2
  delta_right : Outport  Port=3
  tag scope: contact_left=global, contact_nose=global, contact_right=global, delta_left=global, delta_nose=global, delta_right=global
  wires:
  Nose_pos_g/1 -> Selector/1
  Left_pos_g/1 -> Selector1/1
  Right_pos_g/1 -> Selector2/1
  Subtract/1 -> Subtract3/2
  Subtract1/1 -> Subtract4/2
  Subtract2/1 -> Subtract5/2
  Constant/1 -> Subtract5/1, Subtract4/1, Subtract3/1
  Saturation/1 -> Scope/1, delta_nose/1, [delta_nose]
  Saturation1/1 -> [delta_left], delta_left/1, Scope1/1
  Saturation2/1 -> [delta_right], delta_right/1
  Subtract3/1 -> Switch3/2, Saturation/1
  Subtract4/1 -> Switch4/2, Saturation1/1
  Subtract5/1 -> Switch5/2, Saturation2/1
  Constant2/1 -> Switch3/3, Switch5/3, Switch4/3
  Constant4/1 -> Switch5/1, Switch4/1, Switch3/1
  Switch3/1 -> [contact_nose]
  Switch5/1 -> [contact_right]
  Switch4/1 -> [contact_left]
  Constant1/1 -> Subtract/1, Subtract1/1, Subtract2/1
  Selector/1 -> Subtract/2
  Selector1/1 -> Subtract1/2
  Selector2/1 -> Subtract2/2

== system landing_model/control/俯仰通道/俯仰通道/伪攻角回路 ==
  q : Inport
  Integrator : Integrator  ExternalReset=rising
  Product : Product
  Subsystem : Subsystem
  Sum : Sum  Inputs=|+-
  To Workspace : ToWorkspace  VariableName=a34  SaveFormat=Timeseries  SampleTime=-1
  alpha_c : Outport
  wires:
  q/1 -> Sum/1
  Sum/1 -> Integrator/1
  Integrator/1 -> alpha_c/1, Product/2
  Product/1 -> Sum/2
  Subsystem/1(a34) -> Product/1, To Workspace/1
  [fly_height] -> Integrator/2

== system landing_model/control/偏航通道/偏航通道三回路控制/伪攻角回路 ==
  r : Inport
  Integrator : Integrator  ExternalReset=rising
  Product : Product
  Subsystem : Subsystem
  Sum : Sum  Inputs=|+-
  beta_c : Outport
  wires:
  r/1 -> Sum/1
  Sum/1 -> Integrator/1
  Integrator/1 -> beta_c/1, Product/2
  Product/1 -> Sum/2
  Subsystem/1(b) -> Product/1
  [start_fly] -> Integrator/2

== system landing_model/6DOF-MODEL/动力学/起落架模型/三轮在地系下的力/摩擦圆限幅 ==
  N_nose : Inport
  N_left : Inport  Port=2
  N_right : Inport  Port=3
  F_long_nose : Inport  Port=4
  F_long_left : Inport  Port=5
  F_long_right : Inport  Port=6
  F_lat_nose : Inport  Port=7
  F_lat_left : Inport  Port=8
  F_lat_right : Inport  Port=9
  主轮摩擦圆限幅右 : MATLAB Function  TreatAsAtomicUnit=on
  主轮摩擦圆限幅左 : MATLAB Function  TreatAsAtomicUnit=on
  前轮摩擦圆限幅 : MATLAB Function  TreatAsAtomicUnit=on
  F_long_nose_out : Outport
  F_long_left_out : Outport  Port=2
  F_long_right_out : Outport  Port=3
  F_lat__nose_out : Outport  Port=4
  F_lat_left_out : Outport  Port=5
  F_lat_right_out : Outport  Port=6
  wires:
  前轮摩擦圆限幅/1(F_long_out) -> F_long_nose_out/1
  前轮摩擦圆限幅/2(F_lat_out) -> F_lat__nose_out/1
  主轮摩擦圆限幅左/2(F_lat_out) -> F_lat_left_out/1
  主轮摩擦圆限幅左/1(F_long_out) -> F_long_left_out/1
  主轮摩擦圆限幅右/2(F_lat_out) -> F_lat_right_out/1
  主轮摩擦圆限幅右/1(F_long_out) -> F_long_right_out/1
  N_nose/1 -> 前轮摩擦圆限幅/1(N)
  F_long_nose/1 -> 前轮摩擦圆限幅/2(F_long)
  F_lat_nose/1 -> 前轮摩擦圆限幅/3(F_lat)
  F_long_left/1 -> 主轮摩擦圆限幅左/2(F_long)
  N_left/1 -> 主轮摩擦圆限幅左/1(N)
  F_lat_right/1 -> 主轮摩擦圆限幅右/3(F_lat)
  F_lat_left/1 -> 主轮摩擦圆限幅左/3(F_lat)
  F_long_right/1 -> 主轮摩擦圆限幅右/2(F_long)
  N_right/1 -> 主轮摩擦圆限幅右/1(N)
